simulink model "Nonlinear_Motor_Tracking"  (R2017a)
settings: Solver=VariableStepAuto  StartTime=0.0  StopTime=10.0  RelTol=1e-3
model workspace (MAT data in the model file):
  I0 = Simulink.Parameter
  I0.Value = 0.1
  I0.DataType = 'auto'
  I0.Dimensions = [1 1]
  J = Simulink.Parameter
  J.Value = 1.06e-05
  J.DataType = 'auto'
  J.Dimensions = [1 1]
  Kf = Simulink.Parameter
  Kf.Value = 0
  Kf.DataType = 'auto'
  Kf.Dimensions = [1 1]
  Kp = Simulink.Parameter
  Kp.Value = 1.95e-07
  Kp.DataType = 'auto'
  Kp.Dimensions = [1 1]
  Kt = Simulink.Parameter
  Kt.Value = 0.00868
  Kt.DataType = 'auto'
  Kt.Dimensions = [1 1]
  Kv = Simulink.Parameter
  Kv.Value = 115.2
  Kv.DataType = 'auto'
  Kv.Dimensions = [1 1]
  L = Simulink.Parameter
  L.Value = 0.001
  L.DataType = 'auto'
  L.Dimensions = [1 1]
  R = Simulink.Parameter
  R.Value = 0.6
  R.DataType = 'auto'
  R.Dimensions = [1 1]
libraries: simulink x3
settings Model: Creator=yilun  LastModifiedBy=yilun

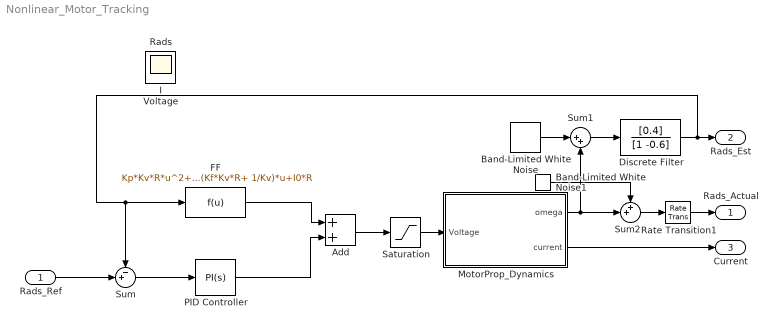
== system Nonlinear_Motor_Tracking ==
  Rads_Ref : Inport
  Add : Sum
  Band-Limited White Noise : simulink/Sources/Band-Limited White Noise  Cov=[0.03]  Ts=0.001  seed=randi(10000,1)
  Band-Limited White Noise1 : simulink/Sources/Band-Limited White Noise  Cov=[0.01]  Ts=0.01  seed=randi(10000,1)
  Discrete Filter : DiscreteFilter  Numerator=[0.4]  Denominator=[1 -0.6]  InitialStates=600
  FF : Fcn  Expr=Kp*Kv*R*u^2+(Kf*Kv*R+ 1/Kv)*u+I0*R
  MotorProp_Dynamics : Subsystem
  PID Controller : simulink/Continuous/PID Controller  Controller=PI  TimeDomain=Continuous-time  SampleTime=-1  IntegratorMethod=Forward Euler  FilterMethod=Forward Euler  Form=Parallel  UseFilter=on  ControllerParametersSource=internal  P=0.065  I=0.2  D=0  N=100  InitialConditionSource=internal  InitialConditionForIntegrator=0  InitialConditionForFilter=0  ExternalReset=none  LimitOutput=on  UpperSaturationLimit=10  LowerSaturationLimit=-10  LinearizeAsGain=on  AntiWindupMode=clamping  Kb=1  TrackingMode=off  Kt=1  PParamMin=[]  PParamMax=[]  IParamMin=[]  IParamMax=[]  DParamMin=[]  DParamMax=[]  NParamMin=[]  NParamMax=[]  KbParamMin=[]  KbParamMax=[]  KtParamMin=[]  KtParamMax=[]  POutMin=[]  POutMax=[]  IOutMin=[]  IOutMax=[]  DOutMin=[]  DOutMax=[]  NOutMin=[]  NOutMax=[]  KbOutMin=[]  KbOutMax=[]  KtOutMin=[]  KtOutMax=[]  IntegratorOutMin=[]  IntegratorOutMax=[]  FilterOutMin=[]  FilterOutMax=[]  SumOutMin=[]  SumOutMax=[]  SumI1OutMin=[]  SumI1OutMax=[]  SumI2OutMin=[]  SumI2OutMax=[]  SumI3OutMin=[]  SumI3OutMax=[]  SumDOutMin=[]  SumDOutMax=[]  SaturationOutMin=[]  SaturationOutMax=[]  IntegratorContinuousStateAttributes=''  IntegratorStateMustResolveToSignalObject=off  IntegratorRTWStateStorageClass=Auto  FilterContinuousStateAttributes=''  FilterStateMustResolveToSignalObject=off  FilterRTWStateStorageClass=Auto  DifferentiatorICPrevScaledInput=0  DifferentiatorOutMin=[]  DifferentiatorOutMax=[]  InitialConditionSetting=State (most efficient)
  Rate Transition1 : RateTransition
  Saturation : Saturate  UpperLimit=14  LowerLimit=1.2
  Sum : Sum  Inputs=-+|
  Sum1 : Sum  Inputs=|++
  Sum2 : Sum  Inputs=++|
  Rads_Actual : Outport
  Rads_Est : Outport  Port=2
  Current : Outport  Port=3
  I : Scope
  Rads : Scope
  Voltage : Scope
  wires:
  Sum/1 -> PID Controller/1
  PID Controller/1 -> Add/2
  FF/1 -> Add/1
  Saturation/1 -> MotorProp_Dynamics/1(Voltage)
  Sum1/1 -> Discrete Filter/1
  Band-Limited White Noise/1 -> Sum1/1
  Rads_Ref/1 -> Sum/2
  Add/1 -> Saturation/1
  Discrete Filter/1 -> Sum/1, FF/1, Rads_Est/1
  MotorProp_Dynamics/1(omega) -> Sum2/2, Sum1/2
  MotorProp_Dynamics/2(current) -> Current/1
  Sum2/1 -> Rate Transition1/1
  Band-Limited White Noise1/1 -> Sum2/1
  Rate Transition1/1 -> Rads_Actual/1

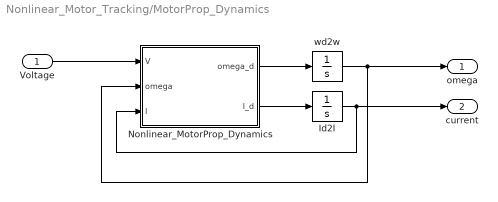
== system Nonlinear_Motor_Tracking/MotorProp_Dynamics ==
  Voltage : Inport
  Id2I : Integrator  InitialCondition=8
  Nonlinear_MotorProp_Dynamics : MATLAB Function  TreatAsAtomicUnit=on
  wd2w : Integrator  InitialCondition=700
  omega : Outport
  current : Outport  Port=2
  wires:
  wd2w/1 -> omega/1, Nonlinear_MotorProp_Dynamics/2(omega)
  Nonlinear_MotorProp_Dynamics/2(I_d) -> Id2I/1
  Id2I/1 -> current/1, Nonlinear_MotorProp_Dynamics/3(I)
  Nonlinear_MotorProp_Dynamics/1(omega_d) -> wd2w/1
  Voltage/1 -> Nonlinear_MotorProp_Dynamics/1(V)

== matlab function Nonlinear_Motor_Tracking/MotorProp_Dynamics/Nonlinear_MotorProp_Dynamics ==
  data: V input; omega_d output; omega input; I input; I_d output; Kp parameter; J parameter; Kf parameter; Kt parameter; I0 parameter; L parameter; Kv parameter; R parameter
function [omega_d, I_d] = fcn(V,omega, I, Kp, J, Kf, Kt, I0, L, Kv, R)
omega_d = (-Kp/J)*(omega^2) - Kf/J*omega + Kt/J*(I-I0);
I_d = 1/L*(-1/Kv*omega - R*I + V);
